simulink model "CORDIC"  (R2021a)
settings: Solver=VariableStepAuto  StartTime=0.0  StopTime=400  RelTol=1e-3
undefined symbols (not defined in the file or in its folder): AXI4, Lite
libraries: hdlBasic x776, xbsIndex_r4 x1
(part 2 of 7)

== system CORDIC/Rotation ==
  In3 : Inport
  In2 : Inport  Port=2
  Constant : hdlBasic/Constant  const=1.0  gui_display_data_type=Fixed-point  arith_type=Signed (2's comp)  n_bits=16  bin_pt=14  preci_type=Single  exp_width=8  frac_width=24  explicit_period=off  period=1  XmcBlockStatus=1  maskContainerNames=tabcontainer1  block_type=constant  block_config=sysgen:Constant_config
  Constant2 : Constant
  Constant3 : Constant  Value=0
  Constant4 : Constant
  Delay : hdlBasic/Delay  rst=off  en=off  latency=1  reg_retiming=off  XmcBlockStatus=1  maskContainerNames=group1  block_type=delay  block_config=sysgen:Delay_config
  Gateway In1 : hdlBasic/Gateway In  gui_display_data_type=Fixed-point  arith_type=Signed (2's comp)  n_bits=16  bin_pt=13  preci_type=Single  exp_width=8  frac_width=24  rows=1  columns=1  quantization="Round  (unbiased: +/- Inf)"  overflow=Saturate  period=1  UseAsADC=off  ADCChannel='1'  interface=None  automatic_assignment=on  address_offset=hex2dec('00')  intf_name=''  intf_description=''  default_value=0  timing_constraint=None  locs_specified=off  LOCs={}  io_standard={}  inherit_from_input=off  hdl_port=on  XmcBlockStatus=1  maskContainerNames=group4  block_type=gatewayin  block_config=sysgen:gateway_in_config  block_width_w=590  block_height_w=620  block_width=640  block_height=850
  Gateway In2 : hdlBasic/Gateway In  gui_display_data_type=Fixed-point  arith_type=Signed (2's comp)  n_bits=16  bin_pt=13  preci_type=Single  exp_width=8  frac_width=24  rows=1  columns=1  quantization="Round  (unbiased: +/- Inf)"  overflow=Saturate  period=1  UseAsADC=off  ADCChannel='1'  interface=None  automatic_assignment=on  address_offset=hex2dec('00')  intf_name=''  intf_description=''  default_value=0  timing_constraint=None  locs_specified=off  LOCs={}  io_standard={}  inherit_from_input=off  hdl_port=on  XmcBlockStatus=1  maskContainerNames=group4  block_type=gatewayin  block_config=sysgen:gateway_in_config  block_width_w=590  block_height_w=620  block_width=640  block_height=850
  Gateway In4 : hdlBasic/Gateway In  gui_display_data_type=Boolean  arith_type=Boolean  n_bits=16  bin_pt=14  preci_type=Single  exp_width=8  frac_width=24  rows=1  columns=1  quantization="Round  (unbiased: +/- Inf)"  overflow=Saturate  period=1  UseAsADC=off  ADCChannel='1'  interface=None  automatic_assignment=on  address_offset=hex2dec('00')  intf_name=''  intf_description=''  default_value=0  timing_constraint=None  locs_specified=off  LOCs={}  io_standard={}  inherit_from_input=off  hdl_port=on  XmcBlockStatus=1  maskContainerNames=group4  block_type=gatewayin  block_config=sysgen:gateway_in_config  block_width_w=590  block_height_w=620  block_width=640  block_height=850
  Gateway In5 : hdlBasic/Gateway In  gui_display_data_type=Boolean  arith_type=Boolean  n_bits=16  bin_pt=14  preci_type=Single  exp_width=8  frac_width=24  rows=1  columns=1  quantization="Round  (unbiased: +/- Inf)"  overflow=Saturate  period=1  UseAsADC=off  ADCChannel='1'  interface=None  automatic_assignment=on  address_offset=hex2dec('00')  intf_name=''  intf_description=''  default_value=0  timing_constraint=None  locs_specified=off  LOCs={}  io_standard={}  inherit_from_input=off  hdl_port=on  XmcBlockStatus=1  maskContainerNames=group4  block_type=gatewayin  block_config=sysgen:gateway_in_config  block_width_w=590  block_height_w=620  block_width=640  block_height=850
  Gateway In6 : hdlBasic/Gateway In  gui_display_data_type=Boolean  arith_type=Boolean  n_bits=16  bin_pt=3  preci_type=Single  exp_width=8  frac_width=24  rows=1  columns=1  quantization="Round  (unbiased: +/- Inf)"  overflow=Saturate  period=1  UseAsADC=off  ADCChannel='1'  interface=None  automatic_assignment=on  address_offset=hex2dec('00')  intf_name=''  intf_description=''  default_value=0  timing_constraint=None  locs_specified=off  LOCs={}  io_standard={}  inherit_from_input=off  hdl_port=on  XmcBlockStatus=1  maskContainerNames=group4  block_type=gatewayin  block_config=sysgen:gateway_in_config  block_width_w=590  block_height_w=620  block_width=640  block_height=850
  Gateway In7 : hdlBasic/Gateway In  gui_display_data_type=Fixed-point  arith_type=Signed (2's comp)  n_bits=16  bin_pt=13  preci_type=Single  exp_width=8  frac_width=24  rows=1  columns=1  quantization="Round  (unbiased: +/- Inf)"  overflow=Saturate  period=1  UseAsADC=off  ADCChannel='1'  interface=None  automatic_assignment=on  address_offset=hex2dec('00')  intf_name=''  intf_description=''  default_value=0  timing_constraint=None  locs_specified=off  LOCs={}  io_standard={}  inherit_from_input=off  hdl_port=on  XmcBlockStatus=1  maskContainerNames=group4  block_type=gatewayin  block_config=sysgen:gateway_in_config  block_width_w=590  block_height_w=620  block_width=640  block_height=850
  Register : hdlBasic/Register  init=0  rst=off  en=off  XmcBlockStatus=1  maskContainerNames=tabcontainer1  block_type=register  block_config=sysgen:Register_config
  Scope : Scope  NumInputPorts=11
  Vitis HLS1 : hdlBasic/Vitis HLS  anytable='C:\ELEC522\jz118\HLS\cordic\solution1'  fast_sim=off  display_datatype=off  rate_propagation_method=Simulink system period  model_file_path=''  latency=1  block_type=vitis_hls
      settings: infoedit=This block allows including C,C++ and SystemC source files in System Generator for DSP designs.
  Out1 : Outport
  Out9 : Outport  Port=2
  wires:
  Constant4/1 -> Gateway In6/1
  Gateway In5/1 -> Vitis HLS1/1
  Constant3/1 -> Gateway In5/1
  Gateway In6/1 -> Vitis HLS1/2
  Vitis HLS1/9 -> Out9/1
  Vitis HLS1/1 -> Scope/1
  Vitis HLS1/2 -> Scope/2
  Vitis HLS1/3 -> Scope/3
  Vitis HLS1/4 -> Scope/4
  Vitis HLS1/5 -> Scope/5
  Vitis HLS1/6 -> Scope/6
  Vitis HLS1/10 -> Scope/8
  Vitis HLS1/8 -> Scope/7
  Vitis HLS1/11 -> Scope/9
  Vitis HLS1/12 -> Scope/10
  Gateway In7/1 -> Vitis HLS1/3
  Register/1 -> Gateway In7/1
  Gateway In1/1 -> Register/1, Vitis HLS1/4
  In2/1 -> Gateway In1/1
  In3/1 -> Gateway In2/1
  Gateway In2/1 -> Delay/1, Vitis HLS1/5
  Delay/1 -> Out1/1
  Vitis HLS1/7 -> Scope/11
  Constant2/1 -> Gateway In4/1
  Gateway In4/1 -> Vitis HLS1/6

== system CORDIC/Rotation1 ==
  In3 : Inport
  In2 : Inport  Port=2
  Constant2 : Constant
  Constant3 : Constant  Value=0
  Constant4 : Constant
  Delay : hdlBasic/Delay  rst=off  en=off  latency=1  reg_retiming=off  XmcBlockStatus=1  maskContainerNames=group1  block_type=delay  block_config=sysgen:Delay_config
  Gateway In1 : hdlBasic/Gateway In  gui_display_data_type=Fixed-point  arith_type=Signed (2's comp)  n_bits=16  bin_pt=13  preci_type=Single  exp_width=8  frac_width=24  rows=1  columns=1  quantization="Round  (unbiased: +/- Inf)"  overflow=Saturate  period=1  UseAsADC=off  ADCChannel='1'  interface=None  automatic_assignment=on  address_offset=hex2dec('00')  intf_name=''  intf_description=''  default_value=0  timing_constraint=None  locs_specified=off  LOCs={}  io_standard={}  inherit_from_input=off  hdl_port=on  XmcBlockStatus=1  maskContainerNames=group4  block_type=gatewayin  block_config=sysgen:gateway_in_config  block_width_w=590  block_height_w=620  block_width=640  block_height=850
  Gateway In2 : hdlBasic/Gateway In  gui_display_data_type=Fixed-point  arith_type=Signed (2's comp)  n_bits=16  bin_pt=13  preci_type=Single  exp_width=8  frac_width=24  rows=1  columns=1  quantization="Round  (unbiased: +/- Inf)"  overflow=Saturate  period=1  UseAsADC=off  ADCChannel='1'  interface=None  automatic_assignment=on  address_offset=hex2dec('00')  intf_name=''  intf_description=''  default_value=0  timing_constraint=None  locs_specified=off  LOCs={}  io_standard={}  inherit_from_input=off  hdl_port=on  XmcBlockStatus=1  maskContainerNames=group4  block_type=gatewayin  block_config=sysgen:gateway_in_config  block_width_w=590  block_height_w=620  block_width=640  block_height=850
  Gateway In4 : hdlBasic/Gateway In  gui_display_data_type=Boolean  arith_type=Boolean  n_bits=16  bin_pt=14  preci_type=Single  exp_width=8  frac_width=24  rows=1  columns=1  quantization="Round  (unbiased: +/- Inf)"  overflow=Saturate  period=1  UseAsADC=off  ADCChannel='1'  interface=None  automatic_assignment=on  address_offset=hex2dec('00')  intf_name=''  intf_description=''  default_value=0  timing_constraint=None  locs_specified=off  LOCs={}  io_standard={}  inherit_from_input=off  hdl_port=on  XmcBlockStatus=1  maskContainerNames=group4  block_type=gatewayin  block_config=sysgen:gateway_in_config  block_width_w=590  block_height_w=620  block_width=640  block_height=850
  Gateway In5 : hdlBasic/Gateway In  gui_display_data_type=Boolean  arith_type=Boolean  n_bits=16  bin_pt=14  preci_type=Single  exp_width=8  frac_width=24  rows=1  columns=1  quantization="Round  (unbiased: +/- Inf)"  overflow=Saturate  period=1  UseAsADC=off  ADCChannel='1'  interface=None  automatic_assignment=on  address_offset=hex2dec('00')  intf_name=''  intf_description=''  default_value=0  timing_constraint=None  locs_specified=off  LOCs={}  io_standard={}  inherit_from_input=off  hdl_port=on  XmcBlockStatus=1  maskContainerNames=group4  block_type=gatewayin  block_config=sysgen:gateway_in_config  block_width_w=590  block_height_w=620  block_width=640  block_height=850
  Gateway In6 : hdlBasic/Gateway In  gui_display_data_type=Boolean  arith_type=Boolean  n_bits=16  bin_pt=3  preci_type=Single  exp_width=8  frac_width=24  rows=1  columns=1  quantization="Round  (unbiased: +/- Inf)"  overflow=Saturate  period=1  UseAsADC=off  ADCChannel='1'  interface=None  automatic_assignment=on  address_offset=hex2dec('00')  intf_name=''  intf_description=''  default_value=0  timing_constraint=None  locs_specified=off  LOCs={}  io_standard={}  inherit_from_input=off  hdl_port=on  XmcBlockStatus=1  maskContainerNames=group4  block_type=gatewayin  block_config=sysgen:gateway_in_config  block_width_w=590  block_height_w=620  block_width=640  block_height=850
  Gateway In7 : hdlBasic/Gateway In  gui_display_data_type=Fixed-point  arith_type=Signed (2's comp)  n_bits=16  bin_pt=13  preci_type=Single  exp_width=8  frac_width=24  rows=1  columns=1  quantization="Round  (unbiased: +/- Inf)"  overflow=Saturate  period=1  UseAsADC=off  ADCChannel='1'  interface=None  automatic_assignment=on  address_offset=hex2dec('00')  intf_name=''  intf_description=''  default_value=0  timing_constraint=None  locs_specified=off  LOCs={}  io_standard={}  inherit_from_input=off  hdl_port=on  XmcBlockStatus=1  maskContainerNames=group4  block_type=gatewayin  block_config=sysgen:gateway_in_config  block_width_w=590  block_height_w=620  block_width=640  block_height=850
  Register : hdlBasic/Register  init=0  rst=off  en=off  XmcBlockStatus=1  maskContainerNames=tabcontainer1  block_type=register  block_config=sysgen:Register_config
  Scope : Scope  NumInputPorts=11
  Vitis HLS1 : hdlBasic/Vitis HLS  anytable='C:\ELEC522\jz118\HLS\cordic\solution1'  fast_sim=off  display_datatype=off  rate_propagation_method=Simulink system period  model_file_path=''  latency=1  block_type=vitis_hls
      settings: infoedit=This block allows including C,C++ and SystemC source files in System Generator for DSP designs.
  Out1 : Outport
  Out9 : Outport  Port=2
  wires:
  Constant4/1 -> Gateway In6/1
  Gateway In5/1 -> Vitis HLS1/1
  Constant3/1 -> Gateway In5/1
  Gateway In6/1 -> Vitis HLS1/2
  Vitis HLS1/9 -> Out9/1
  Vitis HLS1/1 -> Scope/1
  Vitis HLS1/2 -> Scope/2
  Vitis HLS1/3 -> Scope/3
  Vitis HLS1/4 -> Scope/4
  Vitis HLS1/5 -> Scope/5
  Vitis HLS1/6 -> Scope/6
  Vitis HLS1/10 -> Scope/8
  Vitis HLS1/8 -> Scope/7
  Vitis HLS1/11 -> Scope/9
  Vitis HLS1/12 -> Scope/10
  Gateway In7/1 -> Vitis HLS1/3
  Register/1 -> Gateway In7/1
  Gateway In1/1 -> Register/1, Vitis HLS1/4
  In2/1 -> Gateway In1/1
  In3/1 -> Gateway In2/1
  Gateway In2/1 -> Delay/1, Vitis HLS1/5
  Delay/1 -> Out1/1
  Vitis HLS1/7 -> Scope/11
  Constant2/1 -> Gateway In4/1
  Gateway In4/1 -> Vitis HLS1/6

== system CORDIC/Rotation10 ==
  In3 : Inport
  In2 : Inport  Port=2
  Constant : hdlBasic/Constant  const=1.0  gui_display_data_type=Boolean  arith_type=Boolean  n_bits=16  bin_pt=14  preci_type=Single  exp_width=8  frac_width=24  explicit_period=off  period=1  XmcBlockStatus=1  maskContainerNames=tabcontainer1  block_type=constant  block_config=sysgen:Constant_config
  Constant1 : hdlBasic/Constant  const=0  gui_display_data_type=Fixed-point  arith_type=Signed (2's comp)  n_bits=16  bin_pt=13  preci_type=Single  exp_width=8  frac_width=24  explicit_period=off  period=1  XmcBlockStatus=1  maskContainerNames=tabcontainer1  block_type=constant  block_config=sysgen:Constant_config
  Constant3 : hdlBasic/Constant  const=0  gui_display_data_type=Boolean  arith_type=Boolean  n_bits=16  bin_pt=14  preci_type=Single  exp_width=8  frac_width=24  explicit_period=off  period=1  XmcBlockStatus=1  maskContainerNames=tabcontainer1  block_type=constant  block_config=sysgen:Constant_config
  Delay : hdlBasic/Delay  rst=off  en=off  latency=27  reg_retiming=off  XmcBlockStatus=1  maskContainerNames=group1  block_type=delay  block_config=sysgen:Delay_config
  Mux1 : hdlBasic/Mux  inputs=2  en=off  latency=1  precision=Full  arith_type=Unsigned  n_bits=16  bin_pt=14  quantization=Truncate  overflow=Wrap  XmcBlockStatus=1  maskContainerNames=tabcontainer1  block_type=mux  block_config=sysgen:Mux_config
  Terminator{,1..7,16} (9 alike) : Terminator
  Vitis HLS1 : hdlBasic/Vitis HLS  anytable='C:\ELEC522\jz118\HLS\cordic\solution1'  fast_sim=off  display_datatype=off  rate_propagation_method=Simulink system period  model_file_path=''  latency=1  block_type=vitis_hls
      settings: infoedit=This block allows including C,C++ and SystemC source files in System Generator for DSP designs.
  Out1 : Outport
  Out9 : Outport  Port=2
  Out2 : Outport  Port=3
  wires:
  Vitis HLS1/9 -> Out9/1
  In2/1 -> Vitis HLS1/4
  In3/1 -> Delay/1, Vitis HLS1/5
  Delay/1 -> Out1/1
  Constant/1 -> Vitis HLS1/6, Vitis HLS1/2
  Constant1/1 -> Mux1/2
  Vitis HLS1/7 -> Mux1/3
  Vitis HLS1/8 -> Mux1/1
  Mux1/1 -> Out2/1, Vitis HLS1/3
  Constant3/1 -> Vitis HLS1/1
  Vitis HLS1/1 -> Terminator/1
  Vitis HLS1/2 -> Terminator1/1
  Vitis HLS1/3 -> Terminator2/1
  Vitis HLS1/4 -> Terminator3/1
  Vitis HLS1/5 -> Terminator4/1
  Vitis HLS1/6 -> Terminator5/1
  Vitis HLS1/10 -> Terminator6/1
  Vitis HLS1/11 -> Terminator7/1
  Vitis HLS1/12 -> Terminator16/1

== system CORDIC/Rotation11 ==
  In3 : Inport
  In2 : Inport  Port=2
  Constant : hdlBasic/Constant  const=1.0  gui_display_data_type=Boolean  arith_type=Boolean  n_bits=16  bin_pt=14  preci_type=Single  exp_width=8  frac_width=24  explicit_period=off  period=1  XmcBlockStatus=1  maskContainerNames=tabcontainer1  block_type=constant  block_config=sysgen:Constant_config
  Constant1 : hdlBasic/Constant  const=0  gui_display_data_type=Fixed-point  arith_type=Signed (2's comp)  n_bits=16  bin_pt=13  preci_type=Single  exp_width=8  frac_width=24  explicit_period=off  period=1  XmcBlockStatus=1  maskContainerNames=tabcontainer1  block_type=constant  block_config=sysgen:Constant_config
  Constant3 : hdlBasic/Constant  const=0  gui_display_data_type=Boolean  arith_type=Boolean  n_bits=16  bin_pt=14  preci_type=Single  exp_width=8  frac_width=24  explicit_period=off  period=1  XmcBlockStatus=1  maskContainerNames=tabcontainer1  block_type=constant  block_config=sysgen:Constant_config
  Delay : hdlBasic/Delay  rst=off  en=off  latency=27  reg_retiming=off  XmcBlockStatus=1  maskContainerNames=group1  block_type=delay  block_config=sysgen:Delay_config
  Mux1 : hdlBasic/Mux  inputs=2  en=off  latency=1  precision=Full  arith_type=Unsigned  n_bits=16  bin_pt=14  quantization=Truncate  overflow=Wrap  XmcBlockStatus=1  maskContainerNames=tabcontainer1  block_type=mux  block_config=sysgen:Mux_config
  Terminator{,1..7,16} (9 alike) : Terminator
  Vitis HLS1 : hdlBasic/Vitis HLS  anytable='C:\ELEC522\jz118\HLS\cordic\solution1'  fast_sim=off  display_datatype=off  rate_propagation_method=Simulink system period  model_file_path=''  latency=1  block_type=vitis_hls
      settings: infoedit=This block allows including C,C++ and SystemC source files in System Generator for DSP designs.
  Out1 : Outport
  Out9 : Outport  Port=2
  wires:
  Vitis HLS1/9 -> Out9/1
  In2/1 -> Vitis HLS1/4
  In3/1 -> Delay/1, Vitis HLS1/5
  Delay/1 -> Out1/1
  Constant/1 -> Vitis HLS1/6, Vitis HLS1/2
  Constant1/1 -> Mux1/2
  Vitis HLS1/7 -> Mux1/3
  Vitis HLS1/8 -> Mux1/1
  Mux1/1 -> Vitis HLS1/3
  Constant3/1 -> Vitis HLS1/1
  Vitis HLS1/1 -> Terminator/1
  Vitis HLS1/2 -> Terminator1/1
  Vitis HLS1/3 -> Terminator2/1
  Vitis HLS1/4 -> Terminator3/1
  Vitis HLS1/5 -> Terminator4/1
  Vitis HLS1/6 -> Terminator5/1
  Vitis HLS1/10 -> Terminator6/1
  Vitis HLS1/11 -> Terminator7/1
  Vitis HLS1/12 -> Terminator16/1

== system CORDIC/Rotation12 ==
  In3 : Inport
  In2 : Inport  Port=2
  Constant : hdlBasic/Constant  const=1.0  gui_display_data_type=Boolean  arith_type=Boolean  n_bits=16  bin_pt=14  preci_type=Single  exp_width=8  frac_width=24  explicit_period=off  period=1  XmcBlockStatus=1  maskContainerNames=tabcontainer1  block_type=constant  block_config=sysgen:Constant_config
  Constant1 : hdlBasic/Constant  const=0  gui_display_data_type=Fixed-point  arith_type=Signed (2's comp)  n_bits=16  bin_pt=13  preci_type=Single  exp_width=8  frac_width=24  explicit_period=off  period=1  XmcBlockStatus=1  maskContainerNames=tabcontainer1  block_type=constant  block_config=sysgen:Constant_config
  Constant3 : hdlBasic/Constant  const=0  gui_display_data_type=Boolean  arith_type=Boolean  n_bits=16  bin_pt=14  preci_type=Single  exp_width=8  frac_width=24  explicit_period=off  period=1  XmcBlockStatus=1  maskContainerNames=tabcontainer1  block_type=constant  block_config=sysgen:Constant_config
  Delay : hdlBasic/Delay  rst=off  en=off  latency=27  reg_retiming=off  XmcBlockStatus=1  maskContainerNames=group1  block_type=delay  block_config=sysgen:Delay_config
  Mux1 : hdlBasic/Mux  inputs=2  en=off  latency=1  precision=Full  arith_type=Unsigned  n_bits=16  bin_pt=14  quantization=Truncate  overflow=Wrap  XmcBlockStatus=1  maskContainerNames=tabcontainer1  block_type=mux  block_config=sysgen:Mux_config
  Terminator{,1..7,16} (9 alike) : Terminator
  Vitis HLS1 : hdlBasic/Vitis HLS  anytable='C:\ELEC522\jz118\HLS\cordic\solution1'  fast_sim=off  display_datatype=off  rate_propagation_method=Simulink system period  model_file_path=''  latency=1  block_type=vitis_hls
      settings: infoedit=This block allows including C,C++ and SystemC source files in System Generator for DSP designs.
  Out1 : Outport
  Out9 : Outport  Port=2
  wires:
  Vitis HLS1/9 -> Out9/1
  In2/1 -> Vitis HLS1/4
  In3/1 -> Delay/1, Vitis HLS1/5
  Delay/1 -> Out1/1
  Constant/1 -> Vitis HLS1/6, Vitis HLS1/2
  Constant1/1 -> Mux1/2
  Vitis HLS1/7 -> Mux1/3
  Vitis HLS1/8 -> Mux1/1
  Mux1/1 -> Vitis HLS1/3
  Constant3/1 -> Vitis HLS1/1
  Vitis HLS1/1 -> Terminator/1
  Vitis HLS1/2 -> Terminator1/1
  Vitis HLS1/3 -> Terminator2/1
  Vitis HLS1/4 -> Terminator3/1
  Vitis HLS1/5 -> Terminator4/1
  Vitis HLS1/6 -> Terminator5/1
  Vitis HLS1/10 -> Terminator6/1
  Vitis HLS1/11 -> Terminator7/1
  Vitis HLS1/12 -> Terminator16/1

== system CORDIC/Rotation13 ==
  In3 : Inport
  In2 : Inport  Port=2
  Constant : hdlBasic/Constant  const=1.0  gui_display_data_type=Boolean  arith_type=Boolean  n_bits=16  bin_pt=14  preci_type=Single  exp_width=8  frac_width=24  explicit_period=off  period=1  XmcBlockStatus=1  maskContainerNames=tabcontainer1  block_type=constant  block_config=sysgen:Constant_config
  Constant11 : hdlBasic/Constant  const=0  gui_display_data_type=Fixed-point  arith_type=Signed (2's comp)  n_bits=16  bin_pt=13  preci_type=Single  exp_width=8  frac_width=24  explicit_period=off  period=1  XmcBlockStatus=1  maskContainerNames=tabcontainer1  block_type=constant  block_config=sysgen:Constant_config
  Constant3 : hdlBasic/Constant  const=0  gui_display_data_type=Boolean  arith_type=Boolean  n_bits=16  bin_pt=14  preci_type=Single  exp_width=8  frac_width=24  explicit_period=off  period=1  XmcBlockStatus=1  maskContainerNames=tabcontainer1  block_type=constant  block_config=sysgen:Constant_config
  Delay : hdlBasic/Delay  rst=off  en=off  latency=26  reg_retiming=off  XmcBlockStatus=1  maskContainerNames=group1  block_type=delay  block_config=sysgen:Delay_config
  Mux4 : hdlBasic/Mux  inputs=2  en=off  latency=0  precision=Full  arith_type=Unsigned  n_bits=16  bin_pt=14  quantization=Truncate  overflow=Wrap  XmcBlockStatus=1  maskContainerNames=tabcontainer1  block_type=mux  block_config=sysgen:Mux_config
  Register : hdlBasic/Register  init=0  rst=off  en=on  XmcBlockStatus=1  maskContainerNames=tabcontainer1  block_type=register  block_config=sysgen:Register_config
  Scope2 : Scope
  Scope3 : Scope
  Terminator{,1..5,7,16} (8 alike) : Terminator
  Vitis HLS1 : hdlBasic/Vitis HLS  anytable='C:\ELEC522\jz118\HLS\cordic\solution1'  fast_sim=off  display_datatype=off  rate_propagation_method=Simulink system period  model_file_path=''  latency=1  block_type=vitis_hls
      settings: infoedit=This block allows including C,C++ and SystemC source files in System Generator for DSP designs.
  Out1 : Outport
  Out9 : Outport  Port=2
  Out2 : Outport  Port=3
  Out3 : Outport  Port=4
  wires:
  In2/1 -> Scope2/1, Vitis HLS1/4
  In3/1 -> Scope3/1, Delay/1, Vitis HLS1/5
  Delay/1 -> Out1/1
  Constant/1 -> Vitis HLS1/2, Vitis HLS1/6
  Constant3/1 -> Vitis HLS1/1
  Vitis HLS1/1 -> Terminator/1
  Vitis HLS1/2 -> Terminator1/1
  Vitis HLS1/3 -> Terminator2/1
  Vitis HLS1/4 -> Terminator3/1
  Vitis HLS1/5 -> Terminator4/1
  Vitis HLS1/6 -> Terminator5/1
  Vitis HLS1/11 -> Terminator7/1
  Vitis HLS1/12 -> Terminator16/1
  Register/1 -> Out3/1, Out2/1, Vitis HLS1/3
  Vitis HLS1/8 -> Register/2
  Vitis HLS1/7 -> Register/1
  Constant11/1 -> Mux4/2
  Mux4/1 -> Out9/1
  Vitis HLS1/9 -> Mux4/3
  Vitis HLS1/10 -> Mux4/1

== system CORDIC/Rotation14 ==
  In3 : Inport
  In2 : Inport  Port=2
  Constant : hdlBasic/Constant  const=1.0  gui_display_data_type=Boolean  arith_type=Boolean  n_bits=16  bin_pt=14  preci_type=Single  exp_width=8  frac_width=24  explicit_period=off  period=1  XmcBlockStatus=1  maskContainerNames=tabcontainer1  block_type=constant  block_config=sysgen:Constant_config
  Constant1 : hdlBasic/Constant  const=0  gui_display_data_type=Fixed-point  arith_type=Signed (2's comp)  n_bits=16  bin_pt=13  preci_type=Single  exp_width=8  frac_width=24  explicit_period=off  period=1  XmcBlockStatus=1  maskContainerNames=tabcontainer1  block_type=constant  block_config=sysgen:Constant_config
  Constant3 : hdlBasic/Constant  const=0  gui_display_data_type=Boolean  arith_type=Boolean  n_bits=16  bin_pt=14  preci_type=Single  exp_width=8  frac_width=24  explicit_period=off  period=1  XmcBlockStatus=1  maskContainerNames=tabcontainer1  block_type=constant  block_config=sysgen:Constant_config
  Delay : hdlBasic/Delay  rst=off  en=off  latency=1  reg_retiming=off  XmcBlockStatus=1  maskContainerNames=group1  block_type=delay  block_config=sysgen:Delay_config
  Mux1 : hdlBasic/Mux  inputs=2  en=off  latency=1  precision=Full  arith_type=Unsigned  n_bits=16  bin_pt=14  quantization=Truncate  overflow=Wrap  XmcBlockStatus=1  maskContainerNames=tabcontainer1  block_type=mux  block_config=sysgen:Mux_config
  Terminator{,1..7,16} (9 alike) : Terminator
  Vitis HLS1 : hdlBasic/Vitis HLS  anytable='C:\ELEC522\jz118\HLS\cordic\solution1'  fast_sim=off  display_datatype=off  rate_propagation_method=Simulink system period  model_file_path=''  latency=1  block_type=vitis_hls
      settings: infoedit=This block allows including C,C++ and SystemC source files in System Generator for DSP designs.
  Out1 : Outport
  Out9 : Outport  Port=2
  wires:
  Vitis HLS1/9 -> Out9/1
  In2/1 -> Vitis HLS1/4
  In3/1 -> Delay/1, Vitis HLS1/5
  Delay/1 -> Out1/1
  Constant/1 -> Vitis HLS1/6, Vitis HLS1/2
  Constant1/1 -> Mux1/2
  Vitis HLS1/7 -> Mux1/3
  Vitis HLS1/8 -> Mux1/1
  Mux1/1 -> Vitis HLS1/3
  Constant3/1 -> Vitis HLS1/1
  Vitis HLS1/1 -> Terminator/1
  Vitis HLS1/2 -> Terminator1/1
  Vitis HLS1/3 -> Terminator2/1
  Vitis HLS1/4 -> Terminator3/1
  Vitis HLS1/5 -> Terminator4/1
  Vitis HLS1/6 -> Terminator5/1
  Vitis HLS1/10 -> Terminator6/1
  Vitis HLS1/11 -> Terminator7/1
  Vitis HLS1/12 -> Terminator16/1

== system CORDIC/Rotation15 ==
  In3 : Inport
  In2 : Inport  Port=2
  Constant : hdlBasic/Constant  const=1.0  gui_display_data_type=Boolean  arith_type=Boolean  n_bits=16  bin_pt=14  preci_type=Single  exp_width=8  frac_width=24  explicit_period=off  period=1  XmcBlockStatus=1  maskContainerNames=tabcontainer1  block_type=constant  block_config=sysgen:Constant_config
  Constant1 : hdlBasic/Constant  const=0  gui_display_data_type=Fixed-point  arith_type=Signed (2's comp)  n_bits=16  bin_pt=13  preci_type=Single  exp_width=8  frac_width=24  explicit_period=off  period=1  XmcBlockStatus=1  maskContainerNames=tabcontainer1  block_type=constant  block_config=sysgen:Constant_config
  Constant3 : hdlBasic/Constant  const=0  gui_display_data_type=Boolean  arith_type=Boolean  n_bits=16  bin_pt=14  preci_type=Single  exp_width=8  frac_width=24  explicit_period=off  period=1  XmcBlockStatus=1  maskContainerNames=tabcontainer1  block_type=constant  block_config=sysgen:Constant_config
  Delay : hdlBasic/Delay  rst=off  en=off  latency=1  reg_retiming=off  XmcBlockStatus=1  maskContainerNames=group1  block_type=delay  block_config=sysgen:Delay_config
  Mux1 : hdlBasic/Mux  inputs=2  en=off  latency=1  precision=Full  arith_type=Unsigned  n_bits=16  bin_pt=14  quantization=Truncate  overflow=Wrap  XmcBlockStatus=1  maskContainerNames=tabcontainer1  block_type=mux  block_config=sysgen:Mux_config
  Terminator{,1..7,16} (9 alike) : Terminator
  Vitis HLS1 : hdlBasic/Vitis HLS  anytable='C:\ELEC522\jz118\HLS\cordic\solution1'  fast_sim=off  display_datatype=off  rate_propagation_method=Simulink system period  model_file_path=''  latency=1  block_type=vitis_hls
      settings: infoedit=This block allows including C,C++ and SystemC source files in System Generator for DSP designs.
  Out1 : Outport
  Out9 : Outport  Port=2
  wires:
  Vitis HLS1/9 -> Out9/1
  In2/1 -> Vitis HLS1/4
  In3/1 -> Delay/1, Vitis HLS1/5
  Delay/1 -> Out1/1
  Constant/1 -> Vitis HLS1/6, Vitis HLS1/2
  Constant1/1 -> Mux1/2
  Vitis HLS1/7 -> Mux1/3
  Vitis HLS1/8 -> Mux1/1
  Mux1/1 -> Vitis HLS1/3
  Constant3/1 -> Vitis HLS1/1
  Vitis HLS1/1 -> Terminator/1
  Vitis HLS1/2 -> Terminator1/1
  Vitis HLS1/3 -> Terminator2/1
  Vitis HLS1/4 -> Terminator3/1
  Vitis HLS1/5 -> Terminator4/1
  Vitis HLS1/6 -> Terminator5/1
  Vitis HLS1/10 -> Terminator6/1
  Vitis HLS1/11 -> Terminator7/1
  Vitis HLS1/12 -> Terminator16/1

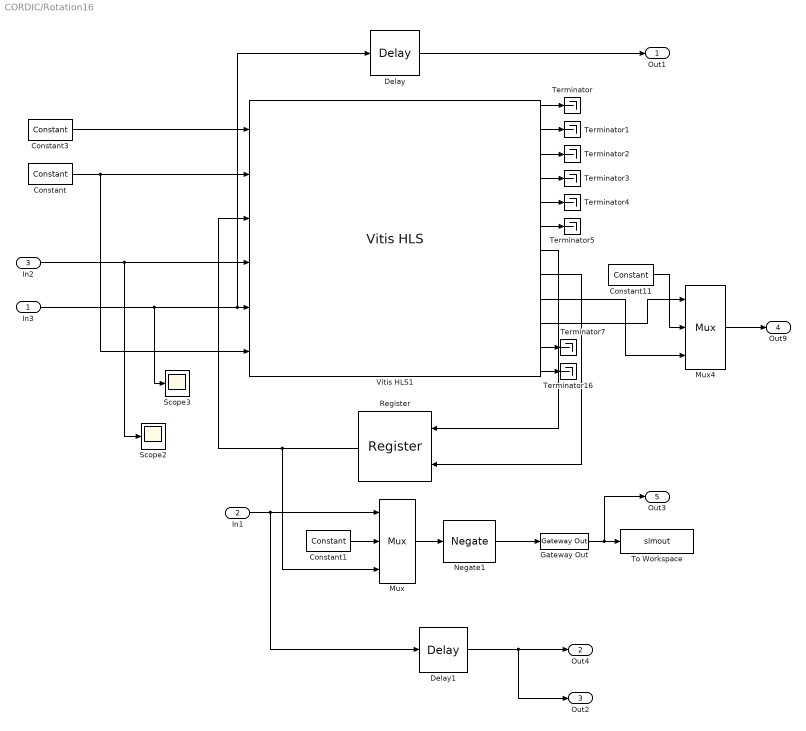
== system CORDIC/Rotation16 ==
  In3 : Inport
  In1 : Inport  Port=2
  In2 : Inport  Port=3
  Constant : hdlBasic/Constant  const=1.0  gui_display_data_type=Boolean  arith_type=Boolean  n_bits=16  bin_pt=14  preci_type=Single  exp_width=8  frac_width=24  explicit_period=off  period=1  XmcBlockStatus=1  maskContainerNames=tabcontainer1  block_type=constant  block_config=sysgen:Constant_config
  Constant1 : hdlBasic/Constant  const=0  gui_display_data_type=Fixed-point  arith_type=Signed (2's comp)  n_bits=16  bin_pt=13  preci_type=Single  exp_width=8  frac_width=24  explicit_period=off  period=1  XmcBlockStatus=1  maskContainerNames=tabcontainer1  block_type=constant  block_config=sysgen:Constant_config
  Constant11 : hdlBasic/Constant  const=0  gui_display_data_type=Fixed-point  arith_type=Signed (2's comp)  n_bits=16  bin_pt=13  preci_type=Single  exp_width=8  frac_width=24  explicit_period=off  period=1  XmcBlockStatus=1  maskContainerNames=tabcontainer1  block_type=constant  block_config=sysgen:Constant_config
  Constant3 : hdlBasic/Constant  const=0  gui_display_data_type=Boolean  arith_type=Boolean  n_bits=16  bin_pt=14  preci_type=Single  exp_width=8  frac_width=24  explicit_period=off  period=1  XmcBlockStatus=1  maskContainerNames=tabcontainer1  block_type=constant  block_config=sysgen:Constant_config
  Delay : hdlBasic/Delay  rst=off  en=off  latency=27  reg_retiming=off  XmcBlockStatus=1  maskContainerNames=group1  block_type=delay  block_config=sysgen:Delay_config
  Delay1 : hdlBasic/Delay  rst=off  en=off  latency=27  reg_retiming=off  XmcBlockStatus=1  maskContainerNames=group1  block_type=delay  block_config=sysgen:Delay_config
  Gateway Out : hdlBasic/Gateway Out  inherit_from_input=off  hdl_port=on  rows=1  columns=1  UseAsDAC=off  DACChannel='1'  interface=None  automatic_assignment=on  address_offset=hex2dec('00')  intf_name=''  intf_description=''  timing_constraint=None  locs_specified=off  LOCs={}  io_standard={}  XmcBlockStatus=1  maskContainerNames=group4  block_type=gatewayout  block_config=sysgen:gateway_out_config  block_width_w=590  block_height_w=620  block_width=620  block_height=750
  Mux : hdlBasic/Mux  inputs=2  en=off  latency=1  precision=Full  arith_type=Unsigned  n_bits=16  bin_pt=14  quantization=Truncate  overflow=Wrap  XmcBlockStatus=1  maskContainerNames=tabcontainer1  block_type=mux  block_config=sysgen:Mux_config
  Mux4 : hdlBasic/Mux  inputs=2  en=off  latency=1  precision=Full  arith_type=Unsigned  n_bits=16  bin_pt=14  quantization=Truncate  overflow=Wrap  XmcBlockStatus=1  maskContainerNames=tabcontainer1  block_type=mux  block_config=sysgen:Mux_config
  Negate1 : hdlBasic/Negate  precision=Full  arith_type=Unsigned  n_bits=16  bin_pt=14  quantization=Truncate  overflow=Wrap  en=off  latency=0  XmcBlockStatus=1  maskContainerNames=tabcontainer1  block_type=negate  block_config=sysgen:Negate_config
  Register : hdlBasic/Register  init=0  rst=off  en=on  XmcBlockStatus=1  maskContainerNames=tabcontainer1  block_type=register  block_config=sysgen:Register_config
  Scope2 : Scope
  Scope3 : Scope
  Terminator{,1..5,7,16} (8 alike) : Terminator
  To Workspace : ToWorkspace  VariableName=simout  SaveFormat=Timeseries  SampleTime=-1
  Vitis HLS1 : hdlBasic/Vitis HLS  anytable='C:\ELEC522\jz118\HLS\cordic\solution1'  fast_sim=off  display_datatype=off  rate_propagation_method=Simulink system period  model_file_path=''  latency=1  block_type=vitis_hls
      settings: infoedit=This block allows including C,C++ and SystemC source files in System Generator for DSP designs.
  Out1 : Outport
  Out4 : Outport  Port=2
  Out2 : Outport  Port=3
  Out9 : Outport  Port=4
  Out3 : Outport  Port=5
  wires:
  In2/1 -> Scope2/1, Vitis HLS1/4
  In3/1 -> Scope3/1, Delay/1, Vitis HLS1/5
  Delay/1 -> Out1/1
  Constant/1 -> Vitis HLS1/2, Vitis HLS1/6
  Constant3/1 -> Vitis HLS1/1
  Vitis HLS1/1 -> Terminator/1
  Vitis HLS1/2 -> Terminator1/1
  Vitis HLS1/3 -> Terminator2/1
  Vitis HLS1/4 -> Terminator3/1
  Vitis HLS1/5 -> Terminator4/1
  Vitis HLS1/6 -> Terminator5/1
  Vitis HLS1/11 -> Terminator7/1
  Vitis HLS1/12 -> Terminator16/1
  Register/1 -> Mux/3, Vitis HLS1/3
  Vitis HLS1/8 -> Register/2
  Vitis HLS1/7 -> Register/1
  Constant11/1 -> Mux4/2
  Mux4/1 -> Out9/1
  Vitis HLS1/9 -> Mux4/3
  Vitis HLS1/10 -> Mux4/1
  In1/1 -> Delay1/1, Mux/1
  Constant1/1 -> Mux/2
  Mux/1 -> Negate1/1
  Negate1/1 -> Gateway Out/1
  Gateway Out/1 -> Out3/1, To Workspace/1
  Delay1/1 -> Out2/1, Out4/1

== system CORDIC/Rotation17 ==
  In3 : Inport
  In1 : Inport  Port=2
  In2 : Inport  Port=3
  Constant : hdlBasic/Constant  const=1.0  gui_display_data_type=Boolean  arith_type=Boolean  n_bits=16  bin_pt=14  preci_type=Single  exp_width=8  frac_width=24  explicit_period=off  period=1  XmcBlockStatus=1  maskContainerNames=tabcontainer1  block_type=constant  block_config=sysgen:Constant_config
  Constant1 : hdlBasic/Constant  const=0  gui_display_data_type=Fixed-point  arith_type=Signed (2's comp)  n_bits=16  bin_pt=13  preci_type=Single  exp_width=8  frac_width=24  explicit_period=off  period=1  XmcBlockStatus=1  maskContainerNames=tabcontainer1  block_type=constant  block_config=sysgen:Constant_config
  Constant11 : hdlBasic/Constant  const=0  gui_display_data_type=Fixed-point  arith_type=Signed (2's comp)  n_bits=16  bin_pt=13  preci_type=Single  exp_width=8  frac_width=24  explicit_period=off  period=1  XmcBlockStatus=1  maskContainerNames=tabcontainer1  block_type=constant  block_config=sysgen:Constant_config
  Constant3 : hdlBasic/Constant  const=0  gui_display_data_type=Boolean  arith_type=Boolean  n_bits=16  bin_pt=14  preci_type=Single  exp_width=8  frac_width=24  explicit_period=off  period=1  XmcBlockStatus=1  maskContainerNames=tabcontainer1  block_type=constant  block_config=sysgen:Constant_config
  Delay : hdlBasic/Delay  rst=off  en=off  latency=27  reg_retiming=off  XmcBlockStatus=1  maskContainerNames=group1  block_type=delay  block_config=sysgen:Delay_config
  Delay1 : hdlBasic/Delay  rst=off  en=off  latency=27  reg_retiming=off  XmcBlockStatus=1  maskContainerNames=group1  block_type=delay  block_config=sysgen:Delay_config
  Gateway Out : hdlBasic/Gateway Out  inherit_from_input=off  hdl_port=on  rows=1  columns=1  UseAsDAC=off  DACChannel='1'  interface=None  automatic_assignment=on  address_offset=hex2dec('00')  intf_name=''  intf_description=''  timing_constraint=None  locs_specified=off  LOCs={}  io_standard={}  XmcBlockStatus=1  maskContainerNames=group4  block_type=gatewayout  block_config=sysgen:gateway_out_config  block_width_w=590  block_height_w=620  block_width=620  block_height=750
  Mux : hdlBasic/Mux  inputs=2  en=off  latency=1  precision=Full  arith_type=Unsigned  n_bits=16  bin_pt=14  quantization=Truncate  overflow=Wrap  XmcBlockStatus=1  maskContainerNames=tabcontainer1  block_type=mux  block_config=sysgen:Mux_config
  Mux4 : hdlBasic/Mux  inputs=2  en=off  latency=1  precision=Full  arith_type=Unsigned  n_bits=16  bin_pt=14  quantization=Truncate  overflow=Wrap  XmcBlockStatus=1  maskContainerNames=tabcontainer1  block_type=mux  block_config=sysgen:Mux_config
  Negate1 : hdlBasic/Negate  precision=Full  arith_type=Unsigned  n_bits=16  bin_pt=14  quantization=Truncate  overflow=Wrap  en=off  latency=0  XmcBlockStatus=1  maskContainerNames=tabcontainer1  block_type=negate  block_config=sysgen:Negate_config
  Register : hdlBasic/Register  init=0  rst=off  en=on  XmcBlockStatus=1  maskContainerNames=tabcontainer1  block_type=register  block_config=sysgen:Register_config
  Scope2 : Scope
  Scope3 : Scope
  Terminator{,1..5,7,16} (8 alike) : Terminator
  To Workspace : ToWorkspace  VariableName=simout  SaveFormat=Timeseries  SampleTime=-1
  Vitis HLS1 : hdlBasic/Vitis HLS  anytable='C:\ELEC522\jz118\HLS\cordic\solution1'  fast_sim=off  display_datatype=off  rate_propagation_method=Simulink system period  model_file_path=''  latency=1  block_type=vitis_hls
      settings: infoedit=This block allows including C,C++ and SystemC source files in System Generator for DSP designs.
  Out1 : Outport
  Out4 : Outport  Port=2
  Out9 : Outport  Port=3
  Out3 : Outport  Port=4
  wires:
  In2/1 -> Scope2/1, Vitis HLS1/4
  In3/1 -> Scope3/1, Delay/1, Vitis HLS1/5
  Delay/1 -> Out1/1
  Constant/1 -> Vitis HLS1/2, Vitis HLS1/6
  Constant3/1 -> Vitis HLS1/1
  Vitis HLS1/1 -> Terminator/1
  Vitis HLS1/2 -> Terminator1/1
  Vitis HLS1/3 -> Terminator2/1
  Vitis HLS1/4 -> Terminator3/1
  Vitis HLS1/5 -> Terminator4/1
  Vitis HLS1/6 -> Terminator5/1
  Vitis HLS1/11 -> Terminator7/1
  Vitis HLS1/12 -> Terminator16/1
  Register/1 -> Mux/3, Vitis HLS1/3
  Vitis HLS1/8 -> Register/2
  Vitis HLS1/7 -> Register/1
  Constant11/1 -> Mux4/2
  Mux4/1 -> Out9/1
  Vitis HLS1/9 -> Mux4/3
  Vitis HLS1/10 -> Mux4/1
  In1/1 -> Delay1/1, Mux/1
  Constant1/1 -> Mux/2
  Mux/1 -> Negate1/1
  Negate1/1 -> Gateway Out/1
  Gateway Out/1 -> Out3/1, To Workspace/1
  Delay1/1 -> Out4/1

== system CORDIC/Rotation18 ==
  In3 : Inport
  In2 : Inport  Port=2
  Constant : hdlBasic/Constant  const=1.0  gui_display_data_type=Boolean  arith_type=Boolean  n_bits=16  bin_pt=14  preci_type=Single  exp_width=8  frac_width=24  explicit_period=off  period=1  XmcBlockStatus=1  maskContainerNames=tabcontainer1  block_type=constant  block_config=sysgen:Constant_config
  Constant11 : hdlBasic/Constant  const=0  gui_display_data_type=Fixed-point  arith_type=Signed (2's comp)  n_bits=16  bin_pt=13  preci_type=Single  exp_width=8  frac_width=24  explicit_period=off  period=1  XmcBlockStatus=1  maskContainerNames=tabcontainer1  block_type=constant  block_config=sysgen:Constant_config
  Constant3 : hdlBasic/Constant  const=0  gui_display_data_type=Boolean  arith_type=Boolean  n_bits=16  bin_pt=14  preci_type=Single  exp_width=8  frac_width=24  explicit_period=off  period=1  XmcBlockStatus=1  maskContainerNames=tabcontainer1  block_type=constant  block_config=sysgen:Constant_config
  Delay : hdlBasic/Delay  rst=off  en=off  latency=27  reg_retiming=off  XmcBlockStatus=1  maskContainerNames=group1  block_type=delay  block_config=sysgen:Delay_config
  Mux4 : hdlBasic/Mux  inputs=2  en=off  latency=1  precision=Full  arith_type=Unsigned  n_bits=16  bin_pt=14  quantization=Truncate  overflow=Wrap  XmcBlockStatus=1  maskContainerNames=tabcontainer1  block_type=mux  block_config=sysgen:Mux_config
  Register : hdlBasic/Register  init=0  rst=off  en=on  XmcBlockStatus=1  maskContainerNames=tabcontainer1  block_type=register  block_config=sysgen:Register_config
  Scope2 : Scope
  Scope3 : Scope
  Terminator{,1..5,7,16} (8 alike) : Terminator
  Vitis HLS1 : hdlBasic/Vitis HLS  anytable='C:\ELEC522\jz118\HLS\cordic\solution1'  fast_sim=off  display_datatype=off  rate_propagation_method=Simulink system period  model_file_path=''  latency=1  block_type=vitis_hls
      settings: infoedit=This block allows including C,C++ and SystemC source files in System Generator for DSP designs.
  Out1 : Outport
  Out9 : Outport  Port=2
  Out2 : Outport  Port=3
  Out3 : Outport  Port=4
  wires:
  In2/1 -> Scope2/1, Vitis HLS1/4
  In3/1 -> Scope3/1, Delay/1, Vitis HLS1/5
  Delay/1 -> Out1/1
  Constant/1 -> Vitis HLS1/2, Vitis HLS1/6
  Constant3/1 -> Vitis HLS1/1
  Vitis HLS1/1 -> Terminator/1
  Vitis HLS1/2 -> Terminator1/1
  Vitis HLS1/3 -> Terminator2/1
  Vitis HLS1/4 -> Terminator3/1
  Vitis HLS1/5 -> Terminator4/1
  Vitis HLS1/6 -> Terminator5/1
  Vitis HLS1/11 -> Terminator7/1
  Vitis HLS1/12 -> Terminator16/1
  Register/1 -> Out3/1, Out2/1, Vitis HLS1/3
  Vitis HLS1/8 -> Register/2
  Vitis HLS1/7 -> Register/1
  Constant11/1 -> Mux4/2
  Mux4/1 -> Out9/1
  Vitis HLS1/9 -> Mux4/3
  Vitis HLS1/10 -> Mux4/1

== system CORDIC/Rotation19 ==
  In3 : Inport
  In2 : Inport  Port=2
  Constant : hdlBasic/Constant  const=1.0  gui_display_data_type=Boolean  arith_type=Boolean  n_bits=16  bin_pt=14  preci_type=Single  exp_width=8  frac_width=24  explicit_period=off  period=1  XmcBlockStatus=1  maskContainerNames=tabcontainer1  block_type=constant  block_config=sysgen:Constant_config
  Constant11 : hdlBasic/Constant  const=0  gui_display_data_type=Fixed-point  arith_type=Signed (2's comp)  n_bits=16  bin_pt=13  preci_type=Single  exp_width=8  frac_width=24  explicit_period=off  period=1  XmcBlockStatus=1  maskContainerNames=tabcontainer1  block_type=constant  block_config=sysgen:Constant_config
  Constant3 : hdlBasic/Constant  const=0  gui_display_data_type=Boolean  arith_type=Boolean  n_bits=16  bin_pt=14  preci_type=Single  exp_width=8  frac_width=24  explicit_period=off  period=1  XmcBlockStatus=1  maskContainerNames=tabcontainer1  block_type=constant  block_config=sysgen:Constant_config
  Delay : hdlBasic/Delay  rst=off  en=off  latency=27  reg_retiming=off  XmcBlockStatus=1  maskContainerNames=group1  block_type=delay  block_config=sysgen:Delay_config
  Mux4 : hdlBasic/Mux  inputs=2  en=off  latency=1  precision=Full  arith_type=Unsigned  n_bits=16  bin_pt=14  quantization=Truncate  overflow=Wrap  XmcBlockStatus=1  maskContainerNames=tabcontainer1  block_type=mux  block_config=sysgen:Mux_config
  Register : hdlBasic/Register  init=0  rst=off  en=on  XmcBlockStatus=1  maskContainerNames=tabcontainer1  block_type=register  block_config=sysgen:Register_config
  Scope2 : Scope
  Scope3 : Scope
  Terminator{,1..5,7,16} (8 alike) : Terminator
  Vitis HLS1 : hdlBasic/Vitis HLS  anytable='C:\ELEC522\jz118\HLS\cordic\solution1'  fast_sim=off  display_datatype=off  rate_propagation_method=Simulink system period  model_file_path=''  latency=1  block_type=vitis_hls
      settings: infoedit=This block allows including C,C++ and SystemC source files in System Generator for DSP designs.
  Out1 : Outport
  Out9 : Outport  Port=2
  Out2 : Outport  Port=3
  Out3 : Outport  Port=4
  wires:
  In2/1 -> Scope2/1, Vitis HLS1/4
  In3/1 -> Scope3/1, Delay/1, Vitis HLS1/5
  Delay/1 -> Out1/1
  Constant/1 -> Vitis HLS1/2, Vitis HLS1/6
  Constant3/1 -> Vitis HLS1/1
  Vitis HLS1/1 -> Terminator/1
  Vitis HLS1/2 -> Terminator1/1
  Vitis HLS1/3 -> Terminator2/1
  Vitis HLS1/4 -> Terminator3/1
  Vitis HLS1/5 -> Terminator4/1
  Vitis HLS1/6 -> Terminator5/1
  Vitis HLS1/11 -> Terminator7/1
  Vitis HLS1/12 -> Terminator16/1
  Register/1 -> Out3/1, Out2/1, Vitis HLS1/3
  Vitis HLS1/8 -> Register/2
  Vitis HLS1/7 -> Register/1
  Constant11/1 -> Mux4/2
  Mux4/1 -> Out9/1
  Vitis HLS1/9 -> Mux4/3
  Vitis HLS1/10 -> Mux4/1

== system CORDIC/Rotation2 ==
  In3 : Inport
  In2 : Inport  Port=2
  Constant2 : Constant
  Constant3 : Constant  Value=0
  Constant4 : Constant
  Delay : hdlBasic/Delay  rst=off  en=off  latency=1  reg_retiming=off  XmcBlockStatus=1  maskContainerNames=group1  block_type=delay  block_config=sysgen:Delay_config
  Gateway In1 : hdlBasic/Gateway In  gui_display_data_type=Fixed-point  arith_type=Signed (2's comp)  n_bits=16  bin_pt=13  preci_type=Single  exp_width=8  frac_width=24  rows=1  columns=1  quantization="Round  (unbiased: +/- Inf)"  overflow=Saturate  period=1  UseAsADC=off  ADCChannel='1'  interface=None  automatic_assignment=on  address_offset=hex2dec('00')  intf_name=''  intf_description=''  default_value=0  timing_constraint=None  locs_specified=off  LOCs={}  io_standard={}  inherit_from_input=off  hdl_port=on  XmcBlockStatus=1  maskContainerNames=group4  block_type=gatewayin  block_config=sysgen:gateway_in_config  block_width_w=590  block_height_w=620  block_width=640  block_height=850
  Gateway In2 : hdlBasic/Gateway In  gui_display_data_type=Fixed-point  arith_type=Signed (2's comp)  n_bits=16  bin_pt=13  preci_type=Single  exp_width=8  frac_width=24  rows=1  columns=1  quantization="Round  (unbiased: +/- Inf)"  overflow=Saturate  period=1  UseAsADC=off  ADCChannel='1'  interface=None  automatic_assignment=on  address_offset=hex2dec('00')  intf_name=''  intf_description=''  default_value=0  timing_constraint=None  locs_specified=off  LOCs={}  io_standard={}  inherit_from_input=off  hdl_port=on  XmcBlockStatus=1  maskContainerNames=group4  block_type=gatewayin  block_config=sysgen:gateway_in_config  block_width_w=590  block_height_w=620  block_width=640  block_height=850
  Gateway In4 : hdlBasic/Gateway In  gui_display_data_type=Boolean  arith_type=Boolean  n_bits=16  bin_pt=14  preci_type=Single  exp_width=8  frac_width=24  rows=1  columns=1  quantization="Round  (unbiased: +/- Inf)"  overflow=Saturate  period=1  UseAsADC=off  ADCChannel='1'  interface=None  automatic_assignment=on  address_offset=hex2dec('00')  intf_name=''  intf_description=''  default_value=0  timing_constraint=None  locs_specified=off  LOCs={}  io_standard={}  inherit_from_input=off  hdl_port=on  XmcBlockStatus=1  maskContainerNames=group4  block_type=gatewayin  block_config=sysgen:gateway_in_config  block_width_w=590  block_height_w=620  block_width=640  block_height=850
  Gateway In5 : hdlBasic/Gateway In  gui_display_data_type=Boolean  arith_type=Boolean  n_bits=16  bin_pt=14  preci_type=Single  exp_width=8  frac_width=24  rows=1  columns=1  quantization="Round  (unbiased: +/- Inf)"  overflow=Saturate  period=1  UseAsADC=off  ADCChannel='1'  interface=None  automatic_assignment=on  address_offset=hex2dec('00')  intf_name=''  intf_description=''  default_value=0  timing_constraint=None  locs_specified=off  LOCs={}  io_standard={}  inherit_from_input=off  hdl_port=on  XmcBlockStatus=1  maskContainerNames=group4  block_type=gatewayin  block_config=sysgen:gateway_in_config  block_width_w=590  block_height_w=620  block_width=640  block_height=850
  Gateway In6 : hdlBasic/Gateway In  gui_display_data_type=Boolean  arith_type=Boolean  n_bits=16  bin_pt=3  preci_type=Single  exp_width=8  frac_width=24  rows=1  columns=1  quantization="Round  (unbiased: +/- Inf)"  overflow=Saturate  period=1  UseAsADC=off  ADCChannel='1'  interface=None  automatic_assignment=on  address_offset=hex2dec('00')  intf_name=''  intf_description=''  default_value=0  timing_constraint=None  locs_specified=off  LOCs={}  io_standard={}  inherit_from_input=off  hdl_port=on  XmcBlockStatus=1  maskContainerNames=group4  block_type=gatewayin  block_config=sysgen:gateway_in_config  block_width_w=590  block_height_w=620  block_width=640  block_height=850
  Gateway In7 : hdlBasic/Gateway In  gui_display_data_type=Fixed-point  arith_type=Signed (2's comp)  n_bits=16  bin_pt=13  preci_type=Single  exp_width=8  frac_width=24  rows=1  columns=1  quantization="Round  (unbiased: +/- Inf)"  overflow=Saturate  period=1  UseAsADC=off  ADCChannel='1'  interface=None  automatic_assignment=on  address_offset=hex2dec('00')  intf_name=''  intf_description=''  default_value=0  timing_constraint=None  locs_specified=off  LOCs={}  io_standard={}  inherit_from_input=off  hdl_port=on  XmcBlockStatus=1  maskContainerNames=group4  block_type=gatewayin  block_config=sysgen:gateway_in_config  block_width_w=590  block_height_w=620  block_width=640  block_height=850
  Register : hdlBasic/Register  init=0  rst=off  en=off  XmcBlockStatus=1  maskContainerNames=tabcontainer1  block_type=register  block_config=sysgen:Register_config
  Scope : Scope  NumInputPorts=11
  Vitis HLS1 : hdlBasic/Vitis HLS  anytable='C:\ELEC522\jz118\HLS\cordic\solution1'  fast_sim=off  display_datatype=off  rate_propagation_method=Simulink system period  model_file_path=''  latency=1  block_type=vitis_hls
      settings: infoedit=This block allows including C,C++ and SystemC source files in System Generator for DSP designs.
  Out1 : Outport
  Out9 : Outport  Port=2
  wires:
  Constant4/1 -> Gateway In6/1
  Gateway In5/1 -> Vitis HLS1/1
  Constant3/1 -> Gateway In5/1
  Gateway In6/1 -> Vitis HLS1/2
  Vitis HLS1/9 -> Out9/1
  Vitis HLS1/1 -> Scope/1
  Vitis HLS1/2 -> Scope/2
  Vitis HLS1/3 -> Scope/3
  Vitis HLS1/4 -> Scope/4
  Vitis HLS1/5 -> Scope/5
  Vitis HLS1/6 -> Scope/6
  Vitis HLS1/10 -> Scope/8
  Vitis HLS1/8 -> Scope/7
  Vitis HLS1/11 -> Scope/9
  Vitis HLS1/12 -> Scope/10
  Gateway In7/1 -> Vitis HLS1/3
  Register/1 -> Gateway In7/1
  Gateway In1/1 -> Register/1, Vitis HLS1/4
  In2/1 -> Gateway In1/1
  In3/1 -> Gateway In2/1
  Gateway In2/1 -> Delay/1, Vitis HLS1/5
  Delay/1 -> Out1/1
  Vitis HLS1/7 -> Scope/11
  Constant2/1 -> Gateway In4/1
  Gateway In4/1 -> Vitis HLS1/6

== system CORDIC/Rotation20 ==
  In3 : Inport
  In2 : Inport  Port=2
  Constant : hdlBasic/Constant  const=1.0  gui_display_data_type=Boolean  arith_type=Boolean  n_bits=16  bin_pt=14  preci_type=Single  exp_width=8  frac_width=24  explicit_period=off  period=1  XmcBlockStatus=1  maskContainerNames=tabcontainer1  block_type=constant  block_config=sysgen:Constant_config
  Constant11 : hdlBasic/Constant  const=0  gui_display_data_type=Fixed-point  arith_type=Signed (2's comp)  n_bits=16  bin_pt=13  preci_type=Single  exp_width=8  frac_width=24  explicit_period=off  period=1  XmcBlockStatus=1  maskContainerNames=tabcontainer1  block_type=constant  block_config=sysgen:Constant_config
  Constant3 : hdlBasic/Constant  const=0  gui_display_data_type=Boolean  arith_type=Boolean  n_bits=16  bin_pt=14  preci_type=Single  exp_width=8  frac_width=24  explicit_period=off  period=1  XmcBlockStatus=1  maskContainerNames=tabcontainer1  block_type=constant  block_config=sysgen:Constant_config
  Delay : hdlBasic/Delay  rst=off  en=off  latency=27  reg_retiming=off  XmcBlockStatus=1  maskContainerNames=group1  block_type=delay  block_config=sysgen:Delay_config
  Mux4 : hdlBasic/Mux  inputs=2  en=off  latency=1  precision=Full  arith_type=Unsigned  n_bits=16  bin_pt=14  quantization=Truncate  overflow=Wrap  XmcBlockStatus=1  maskContainerNames=tabcontainer1  block_type=mux  block_config=sysgen:Mux_config
  Register : hdlBasic/Register  init=0  rst=off  en=on  XmcBlockStatus=1  maskContainerNames=tabcontainer1  block_type=register  block_config=sysgen:Register_config
  Scope : Scope  NumInputPorts=3
  Terminator{,1..5,7,16} (8 alike) : Terminator
  Vitis HLS1 : hdlBasic/Vitis HLS  anytable='C:\ELEC522\jz118\HLS\cordic\solution1'  fast_sim=off  display_datatype=off  rate_propagation_method=Simulink system period  model_file_path=''  latency=1  block_type=vitis_hls
      settings: infoedit=This block allows including C,C++ and SystemC source files in System Generator for DSP designs.
  Out1 : Outport
  Out9 : Outport  Port=2
  Out2 : Outport  Port=3
  Out3 : Outport  Port=4
  wires:
  In2/1 -> Scope/2, Vitis HLS1/4
  In3/1 -> Scope/3, Delay/1, Vitis HLS1/5
  Delay/1 -> Out1/1
  Constant/1 -> Vitis HLS1/2, Vitis HLS1/6
  Constant3/1 -> Vitis HLS1/1
  Vitis HLS1/1 -> Terminator/1
  Vitis HLS1/2 -> Terminator1/1
  Vitis HLS1/3 -> Terminator2/1
  Vitis HLS1/4 -> Terminator3/1
  Vitis HLS1/5 -> Terminator4/1
  Vitis HLS1/6 -> Terminator5/1
  Vitis HLS1/11 -> Terminator7/1
  Vitis HLS1/12 -> Terminator16/1
  Register/1 -> Out3/1, Scope/1, Out2/1, Vitis HLS1/3
  Vitis HLS1/8 -> Register/2
  Vitis HLS1/7 -> Register/1
  Constant11/1 -> Mux4/2
  Mux4/1 -> Out9/1
  Vitis HLS1/9 -> Mux4/3
  Vitis HLS1/10 -> Mux4/1
